simulink model "Stage_2_2_Virtual_CAN_Network"  (R2025a)
settings: Solver=VariableStepAuto  StartTime=0.0  StopTime=10.0  RelTol=1e-3
libraries: canmsglib x2, SignalEditorBlockLib x2, simulink x1
settings Model: Creator=sitam  LastModifiedBy=sitam

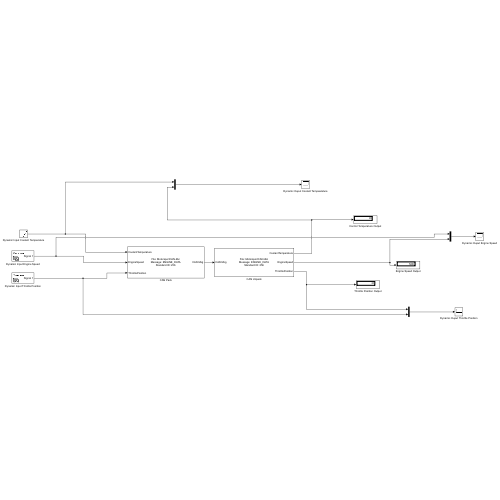
[thumbnail: Simulink's stored preview of the top-level diagram]
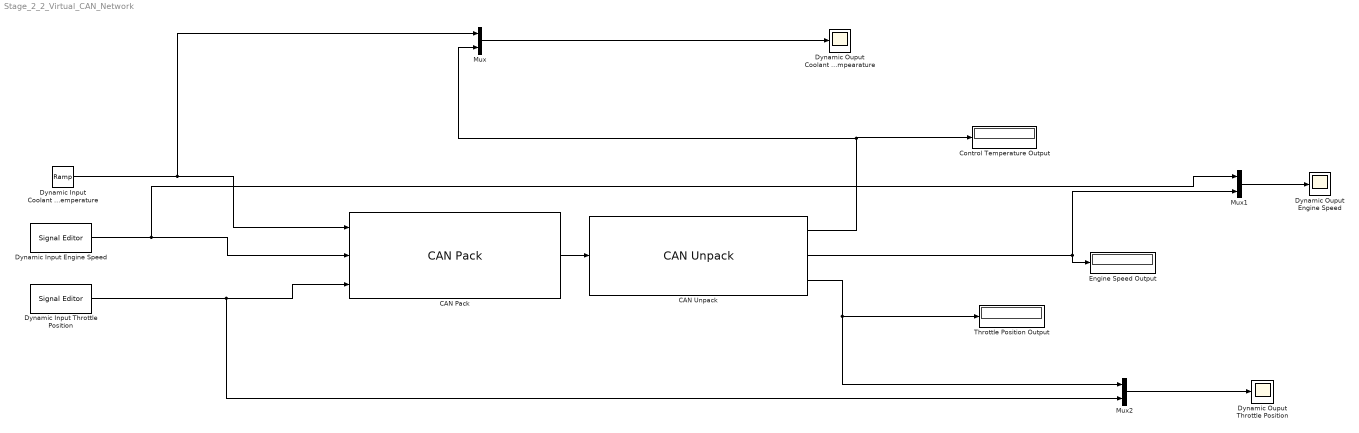
== system Stage_2_2_Virtual_CAN_Network ==
  CAN Pack : canmsglib/CAN Pack  CANdbFile=C:\Users\sitam\OneDrive\Projects\CAN Bus Project\MotorsportCAN.dbc  MsgList=ENGINE_DATA  MsgName=ENGINE_DATA  MsgIDType=Standard (11-bit identifier)  MsgIdentifier=256  CANIDInput=off  MsgLength=8  Remote=off  ApplyMinMax=off  BusOutput=off  SignalInfo={'CoolantTemperature','24','8','LE','unsigned','Standard','0','1','-40','-40','150';'EngineSpeed','0','16','LE','unsigned','Standard','0','0.25','0','0','15000';'ThrottlePosition','16','8','LE','unsigned','Standard','0','0.4','0','0','100'}
      settings: LibrarySourceBlock=canlib/CAN Pack  DataFormat=CANdb specified signals
  CAN Unpack : canmsglib/CAN Unpack  CANdbFile=C:\Users\sitam\OneDrive\Projects\CAN Bus Project\MotorsportCAN.dbc  MsgList=ENGINE_DATA  MsgName=ENGINE_DATA  MsgIDType=Standard (11-bit identifier)  MsgIdentifier=256  MsgLength=8  SignalInfo={'CoolantTemperature','24','8','LE','unsigned','Standard','0','1','-40','-40','150';'EngineSpeed','0','16','LE','unsigned','Standard','0','0.25','0','0','15000';'ThrottlePosition','16','8','LE','unsigned','Standard','0','0.4','0','0','100'}  IDPort=off  TimestampPort=off  ErrorPort=off  RemotePort=off  LengthPort=off  StatusPort=off  ApplyMinMax=off
      settings: LibrarySourceBlock=canlib/CAN Unpack  DataFormat=CANdb specified signals
  Control Temperature Output : Display
  Dynamic Input Coolant Temperature : simulink/Sources/Ramp  slope=1  start=0  InitialOutput=85
  Dynamic Input Engine Speed : SignalEditorBlockLib/Signal Editor  FileName=2_2-enginespeed.mat  ActiveScenario=Scenario  ActiveSignal=Signal 1  IsBus=off  OutputBusObjectStr=Bus: BusObject  SampleTime=0  ZeroCross=off  OutputAfterFinalValue=Setting to zero  Unit=inherit  PreserveSignalName=on  ApplySigPropsToAllScenarios=on  ApplySigPropsToAllSignals=off  SignalPropertySource=Dialog parameters
  Dynamic Input Throttle Position : SignalEditorBlockLib/Signal Editor  FileName=2_2-throttlepos.mat  ActiveScenario=Scenario  ActiveSignal=Signal 1  IsBus=off  OutputBusObjectStr=Bus: BusObject  SampleTime=0  ZeroCross=off  OutputAfterFinalValue=Setting to zero  Unit=inherit  PreserveSignalName=on  ApplySigPropsToAllScenarios=on  ApplySigPropsToAllSignals=off  SignalPropertySource=Dialog parameters
  Dynamic Ouput Coolant Tempearature : Scope
      settings: ActiveDisplayYMinimum=83.75  ActiveDisplayYMaximum=96.25
  Dynamic Ouput Engine Speed : Scope
      settings: ActiveDisplayYMinimum=1875.0000000000002  ActiveDisplayYMaximum=13125  DataLoggingVariableName=ScopeData2
  Dynamic Ouput Throttle Position : Scope
      settings: ActiveDisplayYMinimum=10.000000000000004  ActiveDisplayYMaximum=110
  Engine Speed Output : Display
  Mux : Mux  Inputs=2
  Mux1 : Mux  Inputs=2
  Mux2 : Mux  Inputs=2
  Throttle Position Output : Display
  wires:
  CAN Pack/1 -> CAN Unpack/1
  CAN Unpack/2 -> Engine Speed Output/1, Mux1/2
  CAN Unpack/1 -> Mux/2, Control Temperature Output/1
  CAN Unpack/3 -> Mux2/1, Throttle Position Output/1
  Dynamic Input Coolant Temperature/1 -> Mux/1, CAN Pack/1
  Dynamic Input Engine Speed/1 -> Mux1/1, CAN Pack/2
  Dynamic Input Throttle Position/1 -> Mux2/2, CAN Pack/3
  Mux/1 -> Dynamic Ouput Coolant Tempearature/1
  Mux1/1 -> Dynamic Ouput Engine Speed/1
  Mux2/1 -> Dynamic Ouput Throttle Position/1
